simulink model "series_link_blance_leg"  (R2022b)
settings: Solver=ode45  StartTime=0.0  StopTime=14  MaxStep=0.2  RelTol=1e-3
values from neighbouring files (symbols this model uses):
  a11 = polyfit(leg,k11,2)    [series_get_k.m]
  a12 = polyfit(leg,k12,2)    [series_get_k.m]
  a13 = polyfit(leg,k13,1)    [series_get_k.m]
  a14 = polyfit(leg,k14,2)    [series_get_k.m]
  N = mp*diff(x + L*sin(theta),t,2)    [series_get_k1_length.m]
undefined symbols (not defined in the file or in its folder): X, Y, Z
libraries: sm_lib x74, nesl_utility x17, slpidlib x2, cstblocks x2, matrix_library x2
(part 1 of 3)
settings Model: SimulationMode=accelerator  Creator=Hhop  LastModifiedBy=admin
settings SolverCC: MinimalZcImpactIntegration=on
settings DataIOCC: ReturnWorkspaceOutputs=off
settings DebuggingCC: ReadBeforeWriteMsg=DisableAll  WriteAfterWriteMsg=DisableAll  WriteAfterReadMsg=DisableAll  MultiTaskDSMMsg=none
settings ModelReferenceCC: UpdateModelReferenceTargets=IfOutOfDate
settings SFSimCC: SFSimEcho=off

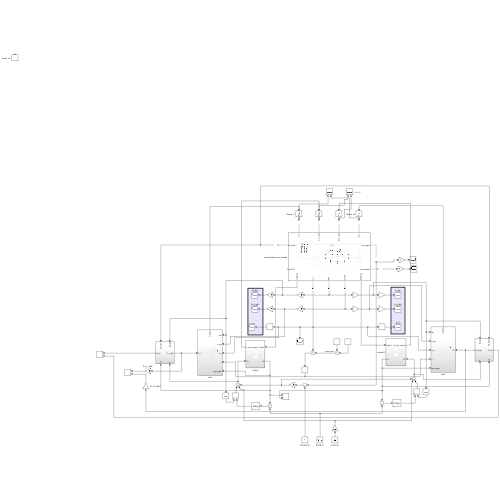
[thumbnail: Simulink's stored preview of the top-level diagram]
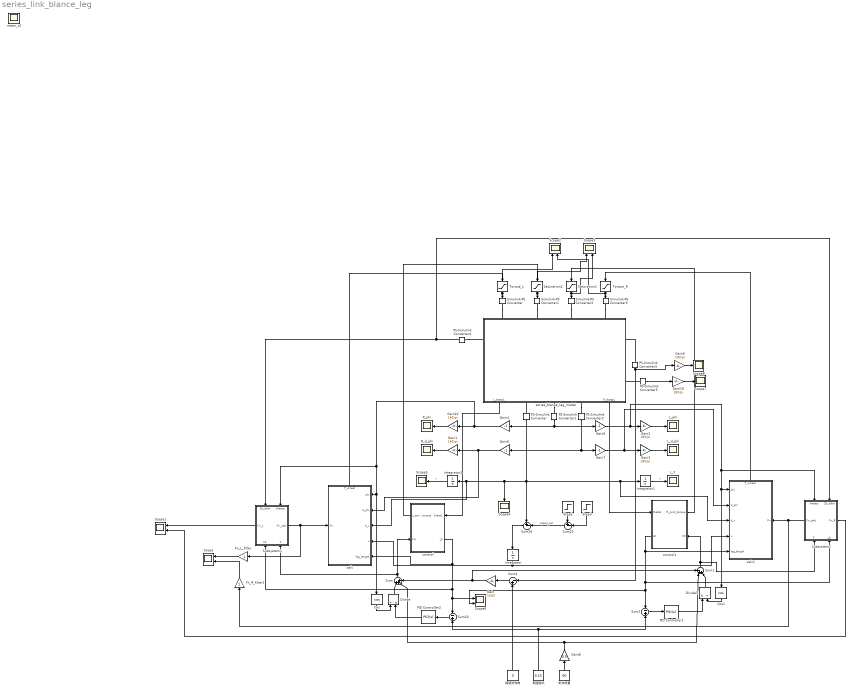
== system series_link_blance_leg ==
  Cos : Trigonometry  Operator=cos
  Cos1 : Trigonometry  Operator=cos
  Divide : Product  Inputs=/*
  Divide1 : Product  Inputs=*/
  Fn_L_filter : Gain
  Fn_R_filter1 : Gain
  Gain : Gain  Gain=-1000
  Gain{1..3,9..10,22} (6 alike) : Gain  Gain=180/pi
  Gain{4..7} (4 alike) : Gain  Gain=-1
  Gain8 : Gain  Gain=0.5
  Integrator : Integrator
  Integrator1 : Integrator
  Integrator2 : Integrator
  L_X : Scope
  L_d_phi : Scope
  L_phi : Scope
  PID Controller1 : slpidlib/PID Controller  Controller=PID  Form=Parallel  TimeDomain=Continuous-time  UseExternalTs=off  SampleTime=-1  IntegratorMethod=Forward Euler  FilterMethod=Forward Euler  ControllerParametersSource=internal  P=600  I=0  UseKiTs=off  D=200  N=100  UseFilter=on  TunerSelectOption=Transfer Function Based (PID Tuner App)  InitialConditionSource=internal  InitialConditionForIntegrator=0  InitialConditionForFilter=0  DifferentiatorICPrevScaledInput=0  ExternalReset=none  TrackingMode=off  Kt=1  LimitOutput=off  SatLimitsSource=internal  UpperSaturationLimit=inf  LowerSaturationLimit=-inf  LinearizeAsGain=on  AntiWindupMode=none  Kb=1  LimitIntegrator=off  UpperIntegratorSaturationLimit=inf  LowerIntegratorSaturationLimit=-inf  POutMin=[]  POutMax=[]  IOutMin=[]  IOutMax=[]  DOutMin=[]  DOutMax=[]  NOutMin=[]  NOutMax=[]  SumOutMin=[]  SumOutMax=[]  SaturationOutMin=[]  SaturationOutMax=[]  PParamMin=[]  PParamMax=[]  IParamMin=[]  IParamMax=[]  DParamMin=[]  DParamMax=[]  NParamMin=[]  NParamMax=[]  KbParamMin=[]  KbParamMax=[]  KtParamMin=[]  KtParamMax=[]  KbOutMin=[]  KbOutMax=[]  KtOutMin=[]  KtOutMax=[]  IntegratorOutMin=[]  IntegratorOutMax=[]  FilterOutMin=[]  FilterOutMax=[]  SumI1OutMin=[]  SumI1OutMax=[]  SumI2OutMin=[]  SumI2OutMax=[]  SumI3OutMin=[]  SumI3OutMax=[]  SumI4OutMin=[]  SumI4OutMax=[]  SumDOutMin=[]  SumDOutMax=[]  DifferentiatorOutMin=[]  DifferentiatorOutMax=[]  FilterDiffOutCoefMin=[]  FilterDiffOutCoefMax=[]  ReciprocalOutMin=[]  ReciprocalOutMax=[]  SumDenOutMin=[]  SumDenOutMax=[]  SumNumOutMin=[]  SumNumOutMax=[]  DivideOutMin=[]  DivideOutMax=[]  UdiffTsProdOutMin=[]  UdiffTsProdOutMax=[]  NTsProdOutMin=[]  NTsProdOutMax=[]  UintegralTsProdOutMin=[]  UintegralTsProdOutMax=[]  UngainTsProdOutMin=[]  UngainTsProdOutMax=[]  ClampingZeroOutDataTypeStr=Inherit: Inherit via back propagation  ClampingZeroOutMin=[]  ClampingZeroOutMax=[]  FilterDenConstantOutDataTypeStr=Inherit: Inherit via back propagation  FilterDenConstantOutMin=[]  FilterDenConstantOutMax=[]  PCopyOutDataTypeStr=Inherit: Inherit via back propagation  PCopyOutMin=[]  PCopyOutMax=[]  NCopyOutDataTypeStr=Inherit: Inherit via back propagation  NCopyOutMin=[]  NCopyOutMax=[]  IntegratorContinuousStateAttributes=''  IntegratorStateMustResolveToSignalObject=off  IntegratorRTWStateStorageClass=Auto  FilterContinuousStateAttributes=''  FilterStateMustResolveToSignalObject=off  FilterRTWStateStorageClass=Auto  ParallelPVariant=InternalParameters  IdealPVariant=Disabled  IVariant=InternalParameters  DVariant=InternalParameters  IntegratorVariant=Continuous  SatVariant=Disabled  AWVariant=Passthrough  PCopyVariant=Disabled  TRVariant=Disabled  FdbkBlocksVariant=Forward  IdealPFdbkVariant=Disabled  SatFdbkVariant=Disabled  DerivativeFilterVariant=ContFilter  NVariant=InternalParameters  NCopyVariant=Disabled  FilterICVariant=InternalICsFilter  IntegratorICVariant=InternalICs  ExternalResetVariant=Disabled  TRSumVariant=Passthrough  SumFdbkVariant=Disabled  SumVariant=Sum_PID  TsampFilterVariant=InternalTs  TsampNgainVariant=Passthrough  TsampIntegralVariant=Passthrough  ExternalSaturationOutDataTypeStr=Inherit: Same as second input
  PID Controller2 : slpidlib/PID Controller  Controller=PID  Form=Parallel  TimeDomain=Continuous-time  UseExternalTs=off  SampleTime=-1  IntegratorMethod=Forward Euler  FilterMethod=Forward Euler  ControllerParametersSource=internal  P=600  I=0  UseKiTs=off  D=200  N=100  UseFilter=on  TunerSelectOption=Transfer Function Based (PID Tuner App)  InitialConditionSource=internal  InitialConditionForIntegrator=0  InitialConditionForFilter=0  DifferentiatorICPrevScaledInput=0  ExternalReset=none  TrackingMode=off  Kt=1  LimitOutput=off  SatLimitsSource=internal  UpperSaturationLimit=inf  LowerSaturationLimit=-inf  LinearizeAsGain=on  AntiWindupMode=none  Kb=1  LimitIntegrator=off  UpperIntegratorSaturationLimit=inf  LowerIntegratorSaturationLimit=-inf  POutMin=[]  POutMax=[]  IOutMin=[]  IOutMax=[]  DOutMin=[]  DOutMax=[]  NOutMin=[]  NOutMax=[]  SumOutMin=[]  SumOutMax=[]  SaturationOutMin=[]  SaturationOutMax=[]  PParamMin=[]  PParamMax=[]  IParamMin=[]  IParamMax=[]  DParamMin=[]  DParamMax=[]  NParamMin=[]  NParamMax=[]  KbParamMin=[]  KbParamMax=[]  KtParamMin=[]  KtParamMax=[]  KbOutMin=[]  KbOutMax=[]  KtOutMin=[]  KtOutMax=[]  IntegratorOutMin=[]  IntegratorOutMax=[]  FilterOutMin=[]  FilterOutMax=[]  SumI1OutMin=[]  SumI1OutMax=[]  SumI2OutMin=[]  SumI2OutMax=[]  SumI3OutMin=[]  SumI3OutMax=[]  SumI4OutMin=[]  SumI4OutMax=[]  SumDOutMin=[]  SumDOutMax=[]  DifferentiatorOutMin=[]  DifferentiatorOutMax=[]  FilterDiffOutCoefMin=[]  FilterDiffOutCoefMax=[]  ReciprocalOutMin=[]  ReciprocalOutMax=[]  SumDenOutMin=[]  SumDenOutMax=[]  SumNumOutMin=[]  SumNumOutMax=[]  DivideOutMin=[]  DivideOutMax=[]  UdiffTsProdOutMin=[]  UdiffTsProdOutMax=[]  NTsProdOutMin=[]  NTsProdOutMax=[]  UintegralTsProdOutMin=[]  UintegralTsProdOutMax=[]  UngainTsProdOutMin=[]  UngainTsProdOutMax=[]  ClampingZeroOutDataTypeStr=Inherit: Inherit via back propagation  ClampingZeroOutMin=[]  ClampingZeroOutMax=[]  FilterDenConstantOutDataTypeStr=Inherit: Inherit via back propagation  FilterDenConstantOutMin=[]  FilterDenConstantOutMax=[]  PCopyOutDataTypeStr=Inherit: Inherit via back propagation  PCopyOutMin=[]  PCopyOutMax=[]  NCopyOutDataTypeStr=Inherit: Inherit via back propagation  NCopyOutMin=[]  NCopyOutMax=[]  IntegratorContinuousStateAttributes=''  IntegratorStateMustResolveToSignalObject=off  IntegratorRTWStateStorageClass=Auto  FilterContinuousStateAttributes=''  FilterStateMustResolveToSignalObject=off  FilterRTWStateStorageClass=Auto  ParallelPVariant=InternalParameters  IdealPVariant=Disabled  IVariant=InternalParameters  DVariant=InternalParameters  IntegratorVariant=Continuous  SatVariant=Disabled  AWVariant=Passthrough  PCopyVariant=Disabled  TRVariant=Disabled  FdbkBlocksVariant=Forward  IdealPFdbkVariant=Disabled  SatFdbkVariant=Disabled  DerivativeFilterVariant=ContFilter  NVariant=InternalParameters  NCopyVariant=Disabled  FilterICVariant=InternalICsFilter  IntegratorICVariant=InternalICs  ExternalResetVariant=Disabled  TRSumVariant=Passthrough  SumFdbkVariant=Disabled  SumVariant=Sum_PID  TsampFilterVariant=InternalTs  TsampNgainVariant=Passthrough  TsampIntegralVariant=Passthrough  ExternalSaturationOutDataTypeStr=Inherit: Same as second input
  PS-Simulink Converter{,1..5} (6 alike) : nesl_utility/PS-Simulink Converter  PhysicalDomain=network_engine_domain  SubClassName=ps_output  LeftPortType=input  RightPortType=output  PseudoPeriodic=off  Frequencies=[]  VectorFormat=inherit  Unit=inherit  AffineConversion=off
  R_d_phi : Scope
  R_phi : Scope
  Saturation1 : Saturate  UpperLimit=45  LowerLimit=-45
  Saturation2 : Saturate  UpperLimit=45  LowerLimit=-45
  Scope{,1..3,6} (5 alike) : Scope  NumInputPorts=2
  Scope{4..5,7..8} (4 alike) : Scope
  Simulink-PS Converter{,1..3} (4 alike) : nesl_utility/Simulink-PS Converter  PhysicalDomain=network_engine_domain  SubClassName=ps_input  LeftPortType=input  RightPortType=output  PseudoPeriodic=off  Frequencies=[]  NoiseDistribution=none  NoiseParameters=[]  Unit=1  AffineConversion=off  FilteringAndDerivatives=provide  SimscapeFilterOrder=1  InputFilterTimeConstant=0.001  UdotUserProvided=0
  Step2 : Step  After=2.5  SampleTime=0
  Step3 : Step  Time=5  After=2.5  SampleTime=0
  Subsystem1 : Subsystem
      settings: PortSchema="{\"entries\":[{\"content\":{\"sides\":[{\"content\":{\"connectorIds\":[\"Out2\"]},\"type\":\"ConnectorPlacement.EquallySpacedRectSide\",\"uuid\":\"45034182-d237-4b20-9dbb-de80031eb49b\"},{\"content\":{\"connectorIds\":[\"Out1\"],\"side\":\"RIGHT\"},\"type\":\"ConnectorPlacement.EquallySpacedRectSide\",\"uuid\":\"39804c16-5df4-48ec-bd6a-84c268544021\"},{\"content\":{\"connectorIds\":[\"In1\",\"In2\"],\"side\":\"TOP\"},\"type\":\"ConnectorPlacement.EquallySpacedRectSide\",\"uuid\":\"bc4ff2f0-88d4-40b7-9830-a63f6eb04eda\"},{\"content\":{\"connectorIds\":[\"In3\",\"In4\"],\"side\":\"BOTTOM\"},\"type\":\"ConnectorPlacement.EquallySpacedRectSide\",\"uuid\":\"f10e4174-89b5-4887-a410-30def43620d9\"}]},\"type\":\"ConnectorPlacement.EquallySpacedConnector\",\"uuid\":\"0f5f2f10-0ef2-4146-8d56-008c67ab6936\"}],\"packageUris\":[\"http://schema.mathworks.com/mf0/Connector/R2020b\"],\"version\":\"1.0\"}"
  Subsystem2 : Subsystem
      settings: PortSchema="{\"entries\":[{\"content\":{\"sides\":[{\"content\":{\"connectorIds\":[\"Out2\"]},\"type\":\"ConnectorPlacement.EquallySpacedRectSide\",\"uuid\":\"45034182-d237-4b20-9dbb-de80031eb49b\"},{\"content\":{\"connectorIds\":[\"Out1\"],\"side\":\"RIGHT\"},\"type\":\"ConnectorPlacement.EquallySpacedRectSide\",\"uuid\":\"39804c16-5df4-48ec-bd6a-84c268544021\"},{\"content\":{\"connectorIds\":[\"In1\",\"In2\"],\"side\":\"TOP\"},\"type\":\"ConnectorPlacement.EquallySpacedRectSide\",\"uuid\":\"bc4ff2f0-88d4-40b7-9830-a63f6eb04eda\"},{\"content\":{\"connectorIds\":[\"In3\",\"In4\"],\"side\":\"BOTTOM\"},\"type\":\"ConnectorPlacement.EquallySpacedRectSide\",\"uuid\":\"f60cc0db-2a5d-4865-8316-be31fea81c9e\"}]},\"type\":\"ConnectorPlacement.EquallySpacedConnector\",\"uuid\":\"0f5f2f10-0ef2-4146-8d56-008c67ab6936\"}],\"packageUris\":[\"http://schema.mathworks.com/mf0/Connector/R2020b\"],\"version\":\"1.0\"}"
  Sum : Sum  Inputs=|+++
  Sum1 : Sum  Inputs=-++|
  Sum2 : Sum  Inputs=-|+
  Sum22 : Sum  Inputs=+-|
  Sum23 : Sum  Inputs=-|+
  Sum26 : Sum  Inputs=+-|
  Sum4 : Sum  Inputs=|-+
  Torque_L : Saturate  UpperLimit=9  LowerLimit=-9
  Torque_R : Saturate  UpperLimit=9  LowerLimit=-9
  calc : Subsystem
      settings: PortSchema="{\"entries\":[{\"content\":{\"sides\":[{\"content\":{\"connectorIds\":[\"In1\",\"In2\",\"In3\",\"In4\",\"In5\"]},\"type\":\"ConnectorPlacement.EquallySpacedRectSide\",\"uuid\":\"055cb80c-cd03-4a8d-aef8-6b3df8c72d3f\"},{\"content\":{\"connectorIds\":[\"In6\"],\"side\":\"RIGHT\"},\"type\":\"ConnectorPlacement.EquallySpacedRectSide\",\"uuid\":\"5756fad1-d70f-4a11-a5af-d2f67bfb0d7e\"},{\"content\":{\"connectorIds\":[\"Out1\"],\"side\":\"TOP\"},\"type\":\"ConnectorPlacement.EquallySpacedRectSide\",\"uuid\":\"9c70cf42-10f8-4525-9406-562484abf580\"}]},\"type\":\"ConnectorPlacement.EquallySpacedConnector\",\"uuid\":\"7084d402-0e44-4d2f-8cc2-1336d196e84d\"}],\"packageUris\":[\"http://schema.mathworks.com/mf0/Connector/R2020b\"],\"version\":\"1.0\"}"
  calc1 : Subsystem
      settings: PortSchema="{\"entries\":[{\"content\":{\"sides\":[{\"content\":{\"connectorIds\":[\"In1\",\"In2\",\"In3\",\"In4\",\"In5\"]},\"type\":\"ConnectorPlacement.EquallySpacedRectSide\",\"uuid\":\"055cb80c-cd03-4a8d-aef8-6b3df8c72d3f\"},{\"content\":{\"connectorIds\":[\"In6\"],\"side\":\"RIGHT\"},\"type\":\"ConnectorPlacement.EquallySpacedRectSide\",\"uuid\":\"5756fad1-d70f-4a11-a5af-d2f67bfb0d7e\"},{\"content\":{\"connectorIds\":[],\"side\":\"TOP\"},\"type\":\"ConnectorPlacement.EquallySpacedRectSide\",\"uuid\":\"9c70cf42-10f8-4525-9406-562484abf580\"},{\"content\":{\"connectorIds\":[\"Out1\"],\"side\":\"BOTTOM\"},\"type\":\"ConnectorPlacement.EquallySpacedRectSide\",\"uuid\":\"92c87742-6ac6-4602-ae8a-30b7231d5549\"}]},\"type\":\"ConnectorPlacement.EquallySpacedConnector\",\"uuid\":\"7084d402-0e44-4d2f-8cc2-1336d196e84d\"}],\"packageUris\":[\"http://schema.mathworks.com/mf0/Connector/R2020b\"],\"version\":\"1.0\"}"
  control : Subsystem
      settings: PortSchema="{\"entries\":[{\"content\":{\"sides\":[{\"content\":{\"connectorIds\":[\"In1\",\"Out2\"]},\"type\":\"ConnectorPlacement.EquallySpacedRectSide\",\"uuid\":\"52f821b9-729d-47ca-ae3d-ba1c6e84da75\"},{\"content\":{\"connectorIds\":[\"Out1\",\"In2\"],\"side\":\"RIGHT\"},\"type\":\"ConnectorPlacement.EquallySpacedRectSide\",\"uuid\":\"ec3ca8e2-1b05-45bc-ab33-c724a2b4f014\"},{\"content\":{\"connectorIds\":[],\"side\":\"TOP\"},\"type\":\"ConnectorPlacement.EquallySpacedRectSide\",\"uuid\":\"0eeea9cd-7beb-490f-b411-de67521f6335\"}]},\"type\":\"ConnectorPlacement.EquallySpacedConnector\",\"uuid\":\"61a91a11-caac-45d5-80d0-d340d78a8d6f\"}],\"packageUris\":[\"http://schema.mathworks.com/mf0/Connector/R2020b\"],\"version\":\"1.0\"}"
  control1 : Subsystem
      settings: PortSchema="{\"entries\":[{\"content\":{\"sides\":[{\"content\":{\"connectorIds\":[\"In1\",\"Out2\"]},\"type\":\"ConnectorPlacement.EquallySpacedRectSide\",\"uuid\":\"52f821b9-729d-47ca-ae3d-ba1c6e84da75\"},{\"content\":{\"connectorIds\":[\"Out1\",\"In2\"],\"side\":\"RIGHT\"},\"type\":\"ConnectorPlacement.EquallySpacedRectSide\",\"uuid\":\"ec3ca8e2-1b05-45bc-ab33-c724a2b4f014\"},{\"content\":{\"connectorIds\":[],\"side\":\"TOP\"},\"type\":\"ConnectorPlacement.EquallySpacedRectSide\",\"uuid\":\"0eeea9cd-7beb-490f-b411-de67521f6335\"}]},\"type\":\"ConnectorPlacement.EquallySpacedConnector\",\"uuid\":\"61a91a11-caac-45d5-80d0-d340d78a8d6f\"}],\"packageUris\":[\"http://schema.mathworks.com/mf0/Connector/R2020b\"],\"version\":\"1.0\"}"
  mean_x2 : Scope
  series_blance_leg_model : Subsystem
      settings: PortSchema="{\"entries\":[{\"content\":{\"sides\":[{\"content\":{\"connectorIds\":[\"LConn1\",\"LConn2\",\"LConn3\",\"LConn4\"]},\"type\":\"ConnectorPlacement.EquallySpacedRectSide\",\"uuid\":\"ed635f35-0836-4900-93e3-56fc3520c8de\"},{\"content\":{\"connectorIds\":[\"Out1\",\"RConn1\",\"RConn2\",\"RConn3\",\"Out2\"],\"side\":\"RIGHT\"},\"type\":\"ConnectorPlacement.EquallySpacedRectSide\",\"uuid\":\"bb235ec0-defd-4ad9-96f6-8533dab3fbd9\"},{\"content\":{\"connectorIds\":[\"LConn5\",\"LConn6\"],\"side\":\"TOP\"},\"type\":\"ConnectorPlacement.EquallySpacedRectSide\",\"uuid\":\"d719db37-8b3a-4344-b330-944fde418334\"},{\"content\":{\"connectorIds\":[\"RConn4\",\"RConn5\"],\"side\":\"BOTTOM\"},\"type\":\"ConnectorPlacement.EquallySpacedRectSide\",\"uuid\":\"20f9270b-6ab1-4e89-bf00-e838d12c3c13\"}]},\"type\":\"ConnectorPlacement.EquallySpacedConnector\",\"uuid\":\"a2f25b71-0047-4a2d-a238-dad76f034ab1\"}],\"packageUris\":[\"http://schema.mathworks.com/mf0/Connector/R2020b\"],\"version\":\"1.0\"}"
  期望滚转角 : Constant  Value=0
  期望腿长 : Constant  Value=0.15
  机体质量 : Constant  Value=60
  wires:
  Integrator2/1 -> Scope5/1  "x"
  Gain22/1 -> R_phi/1
  Gain1/1 -> R_d_phi/1
  Gain3/1 -> L_d_phi/1
  Gain2/1 -> L_phi/1
  Integrator1/1 -> L_X/1  "x"
  control/2(L0) -> Sum23/1, Scope6/1, Subsystem1/4(L0), calc/5(leg_length)
  Sum23/1 -> PID Controller2/1
  control1/2(L0) -> Subsystem2/4(L0), Sum2/1, Scope6/2, calc1/1(leg_length)
  Sum2/1 -> PID Controller1/1
  期望腿长/1 -> Sum23/2, Sum2/2
  机体质量/1 -> Gain8/1
  series_blance_leg_model/1(L_theta1) -> control/1(theta1)
  series_blance_leg_model/2(R_theta1) -> control1/1(theta1)
  PS-Simulink Converter/1 -> calc1/3(d_x), Integrator1/1, Sum26/1, calc/3(d_x), Integrator2/1, Scope4/1
  PS-Simulink Converter1/1 -> Gain4/1, Gain6/1
  PS-Simulink Converter2/1 -> Gain7/1, Gain5/1
  Sum26/1 -> Integrator/1
  Step2/1 -> Sum22/1
  Sum22/1 -> Sum26/2  "speed_set"
  Step3/1 -> Sum22/2
  Integrator/1 -> calc/4(x), calc1/2(x)
  calc1/1(T_wheel) -> Torque_R/1
  Saturation2/1 -> Scope3/1, Simulink-PS Converter1/1
  Saturation1/1 -> Scope3/2, Simulink-PS Converter2/1
  Torque_L/1 -> Scope2/1, Simulink-PS Converter/1
  Torque_R/1 -> Scope2/2, Simulink-PS Converter3/1
  Gain4/1 -> Cos/1, calc/1(phi), Subsystem1/1(thetap), Gain22/1
  Gain5/1 -> calc/2(d_phi), Gain1/1
  Gain6/1 -> Cos1/1, calc1/5(phi), Subsystem2/1(thetap), Gain2/1
  Gain7/1 -> calc1/4(d_phi), Gain3/1
  Gain8/1 -> Sum1/2, Sum/2
  Cos/1 -> Divide/1
  PID Controller2/1 -> Divide/2
  PID Controller1/1 -> Divide1/1
  Cos1/1 -> Divide1/2
  Divide/1 -> Sum/1
  Sum/1 -> control/2(F0), Subsystem1/3(F)
  Gain/1 -> Sum/3, Sum1/1
  Sum1/1 -> control1/2(F0), Subsystem2/3(F)
  Sum4/1 -> Gain/1
  期望滚转角/1 -> Sum4/2
  PS-Simulink Converter3/1 -> Gain9/1, Sum4/1
  Divide1/1 -> Sum1/3
  PS-Simulink Converter4/1 -> Subsystem1/2(Zb_ddot), Subsystem2/2(Zb_ddot)
  Subsystem1/2(Fn_calc) -> Fn_L_filter/1, calc/6(Fn)
  Subsystem2/2(Fn_calc) -> Fn_R_filter1/1, calc1/6(Fn)
  calc/1(T_wheel) -> Torque_L/1
  Fn_L_filter/1 -> Scope/1
  Fn_R_filter1/1 -> Scope/2
  Subsystem1/1(Fn_L) -> Scope1/1
  Subsystem2/1(Fn_R) -> Scope1/2
  control/1(L_joint_torque) -> Saturation2/1
  control1/1(R_joint_torque) -> Saturation1/1
  PS-Simulink Converter5/1 -> Gain10/1
  Gain9/1 -> Scope8/1
  Gain10/1 -> Scope7/1
  connections:
  PS-Simulink Converter/LConn1 -- series_blance_leg_model/RConn1
  series_blance_leg_model/RConn2 -- PS-Simulink Converter1/LConn1
  series_blance_leg_model/RConn3 -- PS-Simulink Converter2/LConn1
  Simulink-PS Converter/RConn1 -- series_blance_leg_model/LConn1
  Simulink-PS Converter1/RConn1 -- series_blance_leg_model/LConn2
  Simulink-PS Converter2/RConn1 -- series_blance_leg_model/LConn3
  Simulink-PS Converter3/RConn1 -- series_blance_leg_model/LConn4
  PS-Simulink Converter3/LConn1 -- series_blance_leg_model/RConn4
  PS-Simulink Converter4/LConn1 -- series_blance_leg_model/LConn5
  PS-Simulink Converter5/LConn1 -- series_blance_leg_model/RConn5

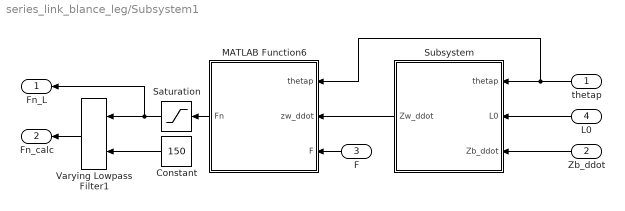
== system series_link_blance_leg/Subsystem1 ==
  thetap : Inport
  Zb_ddot : Inport  Port=2
  F : Inport  Port=3
  L0 : Inport  Port=4
  Constant : Constant  Value=150
  MATLAB Function6 : MATLAB Function  TreatAsAtomicUnit=on
  Saturation : Saturate  UpperLimit=120  LowerLimit=-20  ZeroCross=off
  Subsystem : Subsystem
  Varying Lowpass Filter1 : cstblocks/Linear Parameter Varying/Varying Lowpass Filter  N=2
  Fn_L : Outport
  Fn_calc : Outport  Port=2
  wires:
  Subsystem/1(Zw_ddot) -> MATLAB Function6/2(zw_ddot)
  thetap/1 -> MATLAB Function6/1(thetap), Subsystem/1(thetap)
  F/1 -> MATLAB Function6/3(F)
  Zb_ddot/1 -> Subsystem/3(Zb_ddot)
  L0/1 -> Subsystem/2(L0)
  Constant/1 -> Varying Lowpass Filter1/2
  Saturation/1 -> Fn_L/1, Varying Lowpass Filter1/1
  Varying Lowpass Filter1/1 -> Fn_calc/1
  MATLAB Function6/1(Fn) -> Saturation/1

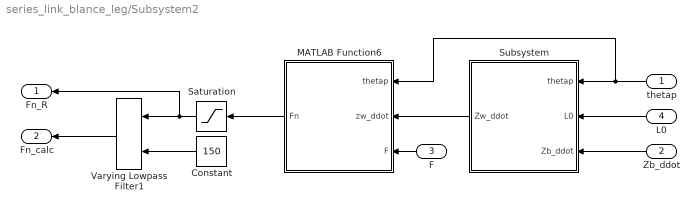
== system series_link_blance_leg/Subsystem2 ==
  thetap : Inport
  Zb_ddot : Inport  Port=2
  F : Inport  Port=3
  L0 : Inport  Port=4
  Constant : Constant  Value=150
  MATLAB Function6 : MATLAB Function  TreatAsAtomicUnit=on
  Saturation : Saturate  UpperLimit=120  LowerLimit=-20  ZeroCross=off
  Subsystem : Subsystem
  Varying Lowpass Filter1 : cstblocks/Linear Parameter Varying/Varying Lowpass Filter  N=2
  Fn_R : Outport
  Fn_calc : Outport  Port=2
  wires:
  L0/1 -> Subsystem/2(L0)
  Zb_ddot/1 -> Subsystem/3(Zb_ddot)
  F/1 -> MATLAB Function6/3(F)
  thetap/1 -> Subsystem/1(thetap), MATLAB Function6/1(thetap)
  Subsystem/1(Zw_ddot) -> MATLAB Function6/2(zw_ddot)
  Saturation/1 -> Fn_R/1, Varying Lowpass Filter1/1
  Constant/1 -> Varying Lowpass Filter1/2
  MATLAB Function6/1(Fn) -> Saturation/1
  Varying Lowpass Filter1/1 -> Fn_calc/1

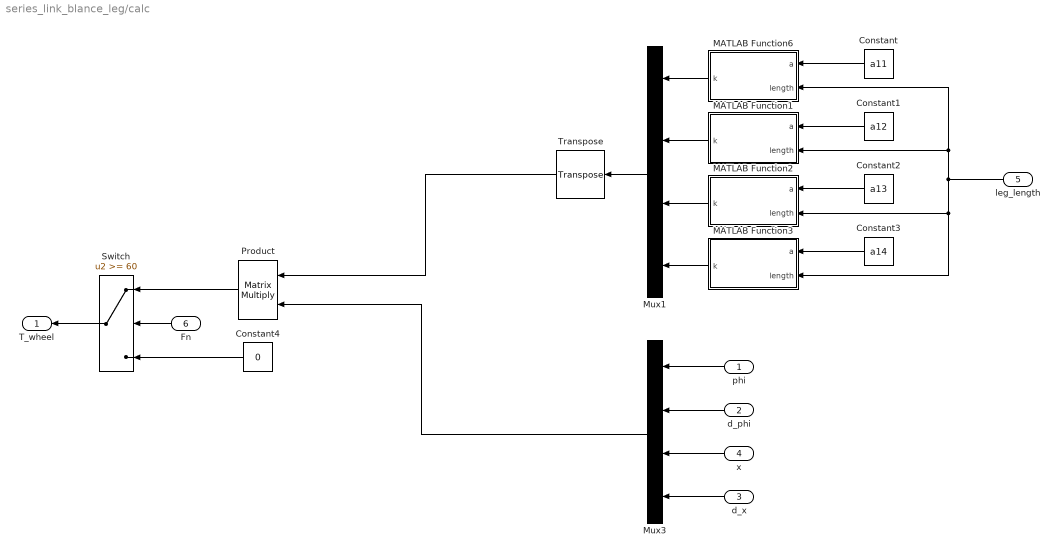
== system series_link_blance_leg/calc ==
  phi : Inport
  d_phi : Inport  Port=2
  d_x : Inport  Port=3
  x : Inport  Port=4
  leg_length : Inport  Port=5
  Fn : Inport  Port=6
  Constant : Constant  Value=a11
  Constant1 : Constant  Value=a12
  Constant2 : Constant  Value=a13
  Constant3 : Constant  Value=a14
  Constant4 : Constant  Value=0
  MATLAB Function1 : MATLAB Function  TreatAsAtomicUnit=on
  MATLAB Function2 : MATLAB Function  TreatAsAtomicUnit=on
  MATLAB Function3 : MATLAB Function  TreatAsAtomicUnit=on
  MATLAB Function6 : MATLAB Function  TreatAsAtomicUnit=on
  Mux1 : Mux
  Mux3 : Mux
  Product : Product  Multiplication=Matrix(*)
  Switch : Switch  Threshold=60  ZeroCross=off  SaturateOnIntegerOverflow=off  InputSameDT=off
  Transpose : matrix_library/Transpose
  T_wheel : Outport
  wires:
  Constant/1 -> MATLAB Function6/1(a)
  Constant1/1 -> MATLAB Function1/1(a)
  Constant2/1 -> MATLAB Function2/1(a)
  Constant3/1 -> MATLAB Function3/1(a)
  leg_length/1 -> MATLAB Function6/2(length), MATLAB Function1/2(length), MATLAB Function3/2(length), MATLAB Function2/2(length)
  d_phi/1 -> Mux3/2
  x/1 -> Mux3/3
  d_x/1 -> Mux3/4
  MATLAB Function6/1(k) -> Mux1/1
  MATLAB Function1/1(k) -> Mux1/2
  MATLAB Function2/1(k) -> Mux1/3
  MATLAB Function3/1(k) -> Mux1/4
  Mux3/1 -> Product/2
  Mux1/1 -> Transpose/1
  Transpose/1 -> Product/1
  Fn/1 -> Switch/2
  Switch/1 -> T_wheel/1
  Product/1 -> Switch/1
  Constant4/1 -> Switch/3
  phi/1 -> Mux3/1

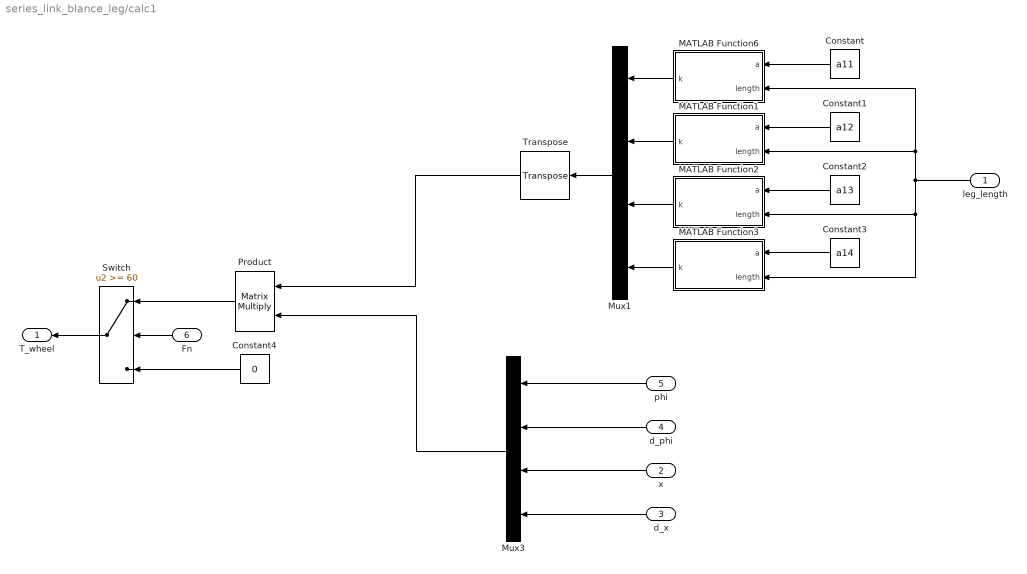
== system series_link_blance_leg/calc1 ==
  leg_length : Inport
  x : Inport  Port=2
  d_x : Inport  Port=3
  d_phi : Inport  Port=4
  phi : Inport  Port=5
  Fn : Inport  Port=6
  Constant : Constant  Value=a11
  Constant1 : Constant  Value=a12
  Constant2 : Constant  Value=a13
  Constant3 : Constant  Value=a14
  Constant4 : Constant  Value=0
  MATLAB Function1 : MATLAB Function  TreatAsAtomicUnit=on
  MATLAB Function2 : MATLAB Function  TreatAsAtomicUnit=on
  MATLAB Function3 : MATLAB Function  TreatAsAtomicUnit=on
  MATLAB Function6 : MATLAB Function  TreatAsAtomicUnit=on
  Mux1 : Mux
  Mux3 : Mux
  Product : Product  Multiplication=Matrix(*)
  Switch : Switch  Threshold=60  ZeroCross=off  SaturateOnIntegerOverflow=off  InputSameDT=off
  Transpose : matrix_library/Transpose
  T_wheel : Outport
  wires:
  d_x/1 -> Mux3/4
  x/1 -> Mux3/3
  d_phi/1 -> Mux3/2
  MATLAB Function1/1(k) -> Mux1/2
  Constant2/1 -> MATLAB Function2/1(a)
  MATLAB Function3/1(k) -> Mux1/4
  MATLAB Function2/1(k) -> Mux1/3
  Constant1/1 -> MATLAB Function1/1(a)
  MATLAB Function6/1(k) -> Mux1/1
  Constant/1 -> MATLAB Function6/1(a)
  Constant3/1 -> MATLAB Function3/1(a)
  Mux3/1 -> Product/2
  Mux1/1 -> Transpose/1
  Transpose/1 -> Product/1
  Fn/1 -> Switch/2
  Constant4/1 -> Switch/3
  Product/1 -> Switch/1
  Switch/1 -> T_wheel/1
  leg_length/1 -> MATLAB Function6/2(length), MATLAB Function1/2(length), MATLAB Function3/2(length), MATLAB Function2/2(length)
  phi/1 -> Mux3/1

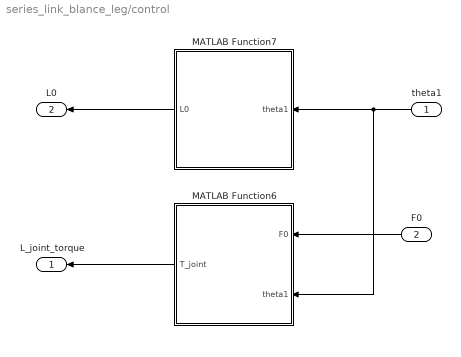
== system series_link_blance_leg/control ==
  theta1 : Inport
  F0 : Inport  Port=2
  MATLAB Function6 : MATLAB Function  TreatAsAtomicUnit=on
  MATLAB Function7 : MATLAB Function  TreatAsAtomicUnit=on
  L_joint_torque : Outport
  L0 : Outport  Port=2
  wires:
  theta1/1 -> MATLAB Function6/2(theta1), MATLAB Function7/1(theta1)
  F0/1 -> MATLAB Function6/1(F0)
  MATLAB Function7/1(L0) -> L0/1
  MATLAB Function6/1(T_joint) -> L_joint_torque/1

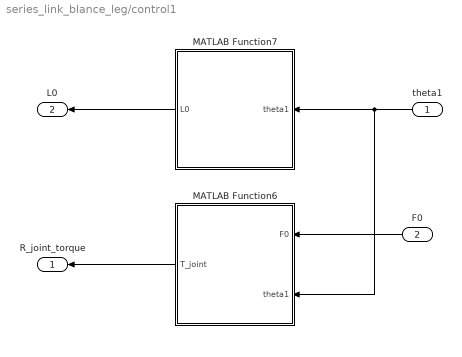
== system series_link_blance_leg/control1 ==
  theta1 : Inport
  F0 : Inport  Port=2
  MATLAB Function6 : MATLAB Function  TreatAsAtomicUnit=on
  MATLAB Function7 : MATLAB Function  TreatAsAtomicUnit=on
  R_joint_torque : Outport
  L0 : Outport  Port=2
  wires:
  MATLAB Function6/1(T_joint) -> R_joint_torque/1
  MATLAB Function7/1(L0) -> L0/1
  F0/1 -> MATLAB Function6/1(F0)
  theta1/1 -> MATLAB Function7/1(theta1), MATLAB Function6/2(theta1)
